simulink model "Simulaciones"  (R2022b)
settings: Solver=VariableStepAuto  StartTime=0.0  StopTime=2  RelTol=1e-3
settings Model: Creator=sebastian  LastModifiedBy=mluser
settings DebuggingCC: UnconnectedInputMsg=warning  UnconnectedOutputMsg=warning  UnconnectedLineMsg=warning
settings ModelReferenceCC: EnableRefExpFcnMdlSchedulingChecks=on
settings RTWCC: DLArmComputeVersion=19.05

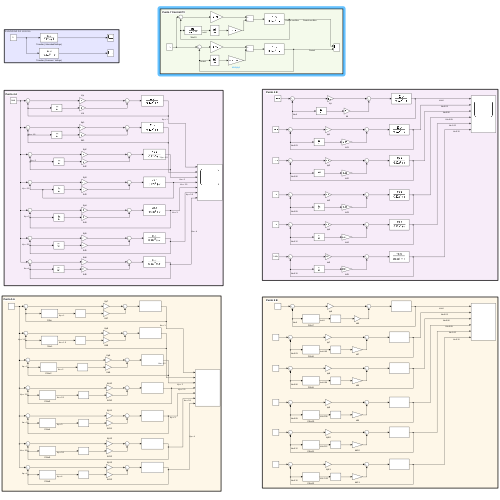
[thumbnail: Simulink's stored preview of the top-level diagram]
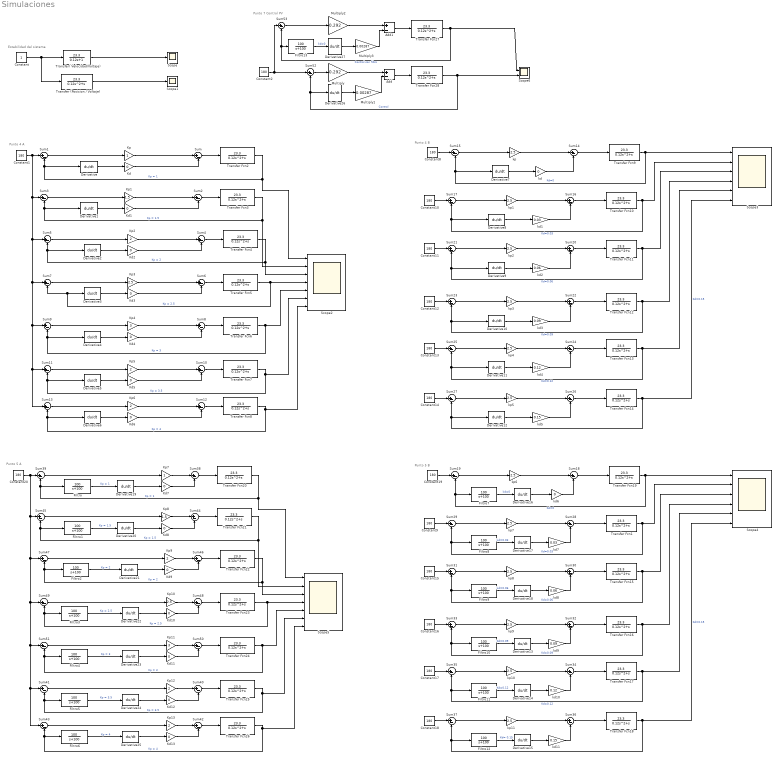
== system Simulaciones ==
  note: Punto 7 Control PV
  note: Punto 4 B
  note: Punto 4 A
  note: Estabilidad del sistema
  note: Punto 5 B
  note: Punto 5 A
  Add : Sum  Inputs=+-
  Add1 : Sum  Inputs=+-
  Constant : Constant
  Constant{1..2,8..20} (15 alike) : Constant  Value=180
  Derivative{,1..27} (28 alike) : Derivative
  Filtro{,1..13} (14 alike) : TransferFcn  Numerator=[100]  Denominator=[ 1 100]
  Kd{,1..13} (14 alike) : Gain  Gain=0
  Kp : Gain
  Kp1 : Gain  Gain=1.5
  Kp10 : Gain  Gain=2.5
  Kp11 : Gain  Gain=3
  Kp{2,5..6,9,12..13} (6 alike) : Gain  Gain=2
  Kp3 : Gain  Gain=2.5
  Kp4 : Gain  Gain=3
  Kp7 : Gain
  Kp8 : Gain  Gain=1.5
  Multiply : Gain  Gain=0.292
  Multiply1 : Gain  Gain=0.00287
  Multiply2 : Gain  Gain=0.292
  Multiply3 : Gain  Gain=0.00287
  Scope : Scope
  Scope1 : Scope
  Scope2 : Scope  NumInputPorts=7
  Scope3 : Scope  NumInputPorts=6
  Scope4 : Scope  NumInputPorts=6
  Scope5 : Scope  NumInputPorts=7
  Scope6 : Scope  NumInputPorts=2
  Sum{,1..53} (54 alike) : Sum  Inputs=|+-
  Transfer (Posicion / Voltaje) : TransferFcn  Numerator=[23.3]  Denominator=[0.12 1 0]
  Transfer Fcn{1..28} (28 alike) : TransferFcn  Numerator=[23.3]  Denominator=[0.12 1 0]
  Transfer( Velocidad/Voltaje) : TransferFcn  Numerator=[23.3]  Denominator=[0.12 1]
  kd : Gain  Gain=0
  kd1 : Gain  Gain=0.03
  kd10 : Gain  Gain=0.12
  kd11 : Gain  Gain=0.15
  kd2 : Gain  Gain=0.06
  kd3 : Gain  Gain=0.09
  kd4 : Gain  Gain=0.12
  kd5 : Gain  Gain=0.15
  kd6 : Gain  Gain=0
  kd7 : Gain  Gain=0.03
  kd8 : Gain  Gain=0.06
  kd9 : Gain  Gain=0.09
  kp{,1..11} (12 alike) : Gain  Gain=2.5
  wires:
  Transfer( Velocidad/Voltaje)/1 -> Scope/1
  Constant/1 -> Transfer (Posicion / Voltaje)/1, Transfer( Velocidad/Voltaje)/1
  Transfer (Posicion / Voltaje)/1 -> Scope1/1
  Derivative/1 -> Kd/1
  Sum1/1 -> Kp/1
  Kp/1 -> Sum/1
  Sum/1 -> Transfer Fcn2/1
  Transfer Fcn2/1 -> Scope2/1, Sum1/2, Derivative/1  "Kp = 1"
  Kd/1 -> Sum/2
  kd/1 -> Sum14/2
  kp/1 -> Sum14/1
  Sum14/1 -> Transfer Fcn9/1
  Sum15/1 -> kp/1
  Transfer Fcn9/1 -> Scope3/1, Derivative7/1, Sum15/2  "Kd=0"
  Derivative7/1 -> kd/1
  Constant8/1 -> Sum15/1
  Sum2/1 -> Transfer Fcn3/1
  Derivative1/1 -> Kd1/1
  Transfer Fcn3/1 -> Sum3/2, Derivative1/1, Scope2/2  "Kp = 1.5"
  Kd1/1 -> Sum2/2
  Sum3/1 -> Kp1/1
  Kp1/1 -> Sum2/1
  Sum4/1 -> Transfer Fcn4/1
  Derivative2/1 -> Kd2/1
  Transfer Fcn4/1 -> Sum5/2, Derivative2/1, Scope2/3  "Kp = 2"
  Kd2/1 -> Sum4/2
  Sum5/1 -> Kp2/1
  Kp2/1 -> Sum4/1
  Derivative3/1 -> Kd3/1
  Sum6/1 -> Transfer Fcn5/1
  Transfer Fcn5/1 -> Sum7/2, Derivative3/1, Scope2/4  "Kp = 2.5"
  Kp3/1 -> Sum6/1
  Sum7/1 -> Kp3/1
  Kd3/1 -> Sum6/2
  Derivative4/1 -> Kd4/1
  Sum8/1 -> Transfer Fcn6/1
  Transfer Fcn6/1 -> Sum9/2, Derivative4/1, Scope2/5  "Kp = 3"
  Kp4/1 -> Sum8/1
  Sum9/1 -> Kp4/1
  Kd4/1 -> Sum8/2
  Derivative5/1 -> Kd5/1
  Sum10/1 -> Transfer Fcn7/1
  Transfer Fcn7/1 -> Scope2/6, Sum11/2, Derivative5/1  "Kp = 3.5"
  Kp5/1 -> Sum10/1
  Sum11/1 -> Kp5/1
  Kd5/1 -> Sum10/2
  Derivative6/1 -> Kd6/1
  Sum12/1 -> Transfer Fcn8/1
  Transfer Fcn8/1 -> Scope2/7, Sum13/2, Derivative6/1  "Kp = 4"
  Constant1/1 -> Sum7/1, Sum13/1, Sum11/1, Sum9/1, Sum5/1, Sum3/1, Sum1/1
  Kp6/1 -> Sum12/1
  Sum13/1 -> Kp6/1
  Kd6/1 -> Sum12/2
  Constant10/1 -> Sum17/1
  kd1/1 -> Sum16/2
  Derivative8/1 -> kd1/1
  kp1/1 -> Sum16/1
  Sum16/1 -> Transfer Fcn10/1
  Transfer Fcn10/1 -> Scope3/2, Derivative8/1, Sum17/2  "Kd=0.03"
  Sum17/1 -> kp1/1
  Constant11/1 -> Sum21/1
  kd2/1 -> Sum20/2
  Derivative9/1 -> kd2/1
  kp2/1 -> Sum20/1
  Sum20/1 -> Transfer Fcn11/1
  Transfer Fcn11/1 -> Scope3/3, Derivative9/1, Sum21/2  "Kd=0.06"
  Sum21/1 -> kp2/1
  Constant12/1 -> Sum23/1
  kd3/1 -> Sum22/2
  Derivative10/1 -> kd3/1
  kp3/1 -> Sum22/1
  Sum22/1 -> Transfer Fcn12/1
  Transfer Fcn12/1 -> Scope3/4, Derivative10/1, Sum23/2  "Kd=0.09"
  Sum23/1 -> kp3/1
  Constant13/1 -> Sum25/1
  kd4/1 -> Sum24/2
  Derivative11/1 -> kd4/1
  kp4/1 -> Sum24/1
  Sum24/1 -> Transfer Fcn13/1
  Transfer Fcn13/1 -> Scope3/5, Derivative11/1, Sum25/2  "Kd=0.12"
  Sum25/1 -> kp4/1
  Constant14/1 -> Sum27/1
  kd5/1 -> Sum26/2
  Derivative12/1 -> kd5/1
  kp5/1 -> Sum26/1
  Sum26/1 -> Transfer Fcn14/1
  Transfer Fcn14/1 -> Scope3/6, Derivative12/1, Sum27/2  "Kd=0.15"
  Sum27/1 -> kp5/1
  Derivative18/1 -> kd8/1
  Derivative16/1 -> kd6/1
  Sum19/1 -> kp6/1
  Sum30/1 -> Transfer Fcn15/1
  kd9/1 -> Sum32/2
  Sum34/1 -> Transfer Fcn17/1
  kd8/1 -> Sum30/2
  kp7/1 -> Sum28/1
  Derivative17/1 -> kd7/1
  Constant9/1 -> Sum29/1
  kd6/1 -> Sum18/2
  kd11/1 -> Sum36/2
  Sum35/1 -> kp10/1
  Sum29/1 -> kp7/1
  Sum32/1 -> Transfer Fcn16/1
  Sum33/1 -> kp9/1
  Constant18/1 -> Sum37/1
  Derivative13/1 -> kd9/1
  kd7/1 -> Sum28/2
  Derivative14/1 -> kd10/1
  Constant19/1 -> Sum19/1
  Sum37/1 -> kp11/1
  Sum18/1 -> Transfer Fcn19/1
  Sum28/1 -> Transfer Fcn1/1
  kd10/1 -> Sum34/2
  kp6/1 -> Sum18/1
  Transfer Fcn16/1 -> Scope4/4, Filtro10/1, Sum33/2  "Kd=0.09"
  Transfer Fcn18/1 -> Scope4/6, Sum37/2, Filtro12/1  "Kd=0.15"
  kp10/1 -> Sum34/1
  Sum36/1 -> Transfer Fcn18/1
  kp8/1 -> Sum30/1
  Sum31/1 -> kp8/1
  Constant17/1 -> Sum35/1
  Transfer Fcn17/1 -> Scope4/5, Filtro11/1, Sum35/2  "Kd=0.12"
  Transfer Fcn19/1 -> Scope4/1, Filtro7/1, Sum19/2  "Kd=0"
  kp9/1 -> Sum32/1
  kp11/1 -> Sum36/1
  Constant15/1 -> Sum31/1
  Derivative15/1 -> kd11/1
  Transfer Fcn1/1 -> Scope4/2, Filtro8/1, Sum29/2  "Kd=0.03"
  Constant16/1 -> Sum33/1
  Transfer Fcn15/1 -> Scope4/3, Filtro9/1, Sum31/2  "Kd=0.06"
  Sum46/1 -> Transfer Fcn22/1
  Sum42/1 -> Transfer Fcn26/1
  Kp8/1 -> Sum44/1
  Sum47/1 -> Kp9/1
  Kp11/1 -> Sum50/1
  Derivative22/1 -> Kd10/1
  Sum45/1 -> Kp8/1
  Derivative24/1 -> Kd12/1
  Transfer Fcn22/1 -> Sum47/2, Filtro2/1, Scope5/3  "Kp = 2"
  Transfer Fcn21/1 -> Sum45/2, Filtro1/1, Scope5/2  "Kp = 1.5"
  Sum51/1 -> Kp11/1
  Derivative20/1 -> Kd8/1
  Kd11/1 -> Sum50/2
  Kp12/1 -> Sum40/1
  Kd9/1 -> Sum46/2
  Kp9/1 -> Sum46/1
  Sum49/1 -> Kp10/1
  Sum48/1 -> Transfer Fcn23/1
  Kp10/1 -> Sum48/1
  Sum38/1 -> Transfer Fcn20/1
  Sum41/1 -> Kp12/1
  Sum40/1 -> Transfer Fcn25/1
  Sum50/1 -> Transfer Fcn24/1
  Kd8/1 -> Sum44/2
  Transfer Fcn25/1 -> Scope5/6, Sum41/2, Filtro5/1  "Kp = 3.5"
  Derivative19/1 -> Kd7/1
  Kd12/1 -> Sum40/2
  Derivative21/1 -> Kd9/1
  Kp7/1 -> Sum38/1
  Kd13/1 -> Sum42/2
  Sum39/1 -> Kp7/1
  Derivative25/1 -> Kd13/1
  Constant20/1 -> Sum49/1, Sum43/1, Sum41/1, Sum51/1, Sum47/1, Sum45/1, Sum39/1
  Sum44/1 -> Transfer Fcn21/1
  Transfer Fcn20/1 -> Scope5/1, Sum39/2, Filtro/1  "Kp = 1"
  Kd10/1 -> Sum48/2
  Kd7/1 -> Sum38/2
  Derivative23/1 -> Kd11/1
  Transfer Fcn24/1 -> Sum51/2, Filtro4/1, Scope5/5  "Kp = 3"
  Kp13/1 -> Sum42/1
  Sum43/1 -> Kp13/1
  Transfer Fcn23/1 -> Sum49/2, Filtro3/1, Scope5/4  "Kp = 2.5"
  Transfer Fcn26/1 -> Scope5/7, Sum43/2, Filtro6/1  "Kp = 4"
  Filtro/1 -> Derivative19/1  "Kp = 1"
  Filtro1/1 -> Derivative20/1  "Kp = 1.5"
  Filtro2/1 -> Derivative21/1  "Kp = 2"
  Filtro3/1 -> Derivative22/1  "Kp = 2.5"
  Filtro4/1 -> Derivative23/1  "Kp = 3"
  Filtro5/1 -> Derivative24/1  "Kp = 3.5"
  Filtro6/1 -> Derivative25/1  "Kp = 4"
  Filtro7/1 -> Derivative16/1  "kd=0"
  Filtro8/1 -> Derivative17/1  "kd=0.03"
  Filtro9/1 -> Derivative18/1  "kd=0.06"
  Filtro10/1 -> Derivative13/1  "Kd=0.09"
  Filtro11/1 -> Derivative14/1  "Kd=0.12"
  Filtro12/1 -> Derivative15/1  "Kd= 0.15"
  Add/1 -> Transfer Fcn28/1
  Derivative26/1 -> Multiply1/1
  Multiply/1 -> Add/1
  Transfer Fcn28/1 -> Derivative26/1, Sum52/2, Scope6/2  "Control"
  Sum52/1 -> Multiply/1
  Constant2/1 -> Sum53/1, Sum52/1
  Multiply1/1 -> Add/2
  Derivative27/1 -> Multiply3/1
  Multiply2/1 -> Add1/1
  Transfer Fcn27/1 -> Filtro13/1, Sum53/2, Scope6/1  "Control con filtro"
  Sum53/1 -> Multiply2/1
  Multiply3/1 -> Add1/2
  Add1/1 -> Transfer Fcn27/1
  Filtro13/1 -> Derivative27/1  "kd=0"
